simulink model "A4_1A_Greenhouse_Moisture_Control_OnOff"  (R2020a)
settings: Solver=VariableStepAuto  StartTime=0.0  StopTime=1000  RelTol=1e-3
settings Model: Creator=mitch  LastModifiedBy=mitch

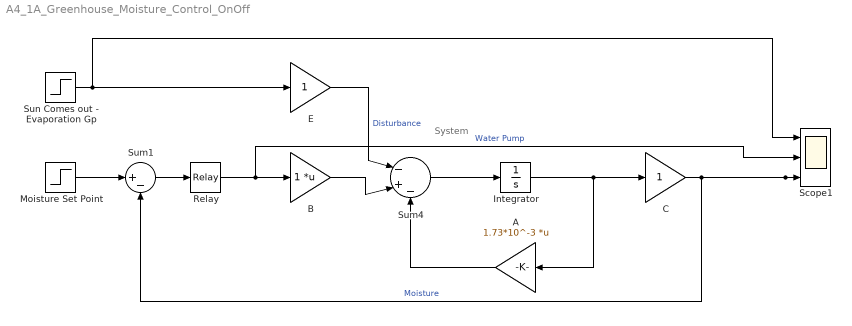
== system A4_1A_Greenhouse_Moisture_Control_OnOff ==
  note: System
  A : Gain  Gain=1.73*10^-3  Multiplication=Matrix(K*u)
  B : Gain  Multiplication=Matrix(K*u)
  C : Gain
  E : Gain
  Integrator : Integrator  InitialCondition=150  LimitOutput=on  UpperSaturationLimit=500  LowerSaturationLimit=0
  Moisture Set Point : Step  Time=100  After=290  SampleTime=0
  Relay : Relay  OnSwitchValue=25  OffSwitchValue=-25  OnOutputValue=5  OutMax=[5]
  Scope1 : Scope  NumInputPorts=3
  Sum1 : Sum  Inputs=|+-
  Sum4 : Sum  Inputs=|-+-
  Sun Comes out - Evaporation Gp : Step  Time=600  SampleTime=0
  wires:
  B/1 -> Sum4/2
  Sun Comes out - Evaporation Gp/1 -> E/1, Scope1/1
  E/1 -> Sum4/1  "Disturbance"
  Sum4/1 -> Integrator/1
  Integrator/1 -> C/1, A/1
  A/1 -> Sum4/3
  C/1 -> Sum1/2, Scope1/3  "Moisture"
  Moisture Set Point/1 -> Sum1/1
  Sum1/1 -> Relay/1
  Relay/1 -> Scope1/2, B/1  "Water Pump"
